simulink model "PX02s"  (R2015b)
settings: Solver=VariableStepAuto  StartTime=0.0  StopTime=10.0  RelTol=1e-3
libraries: fl_lib x10, nesl_utility x3
settings Model: Creator=xmax1946  LastModifiedBy=xmax1946

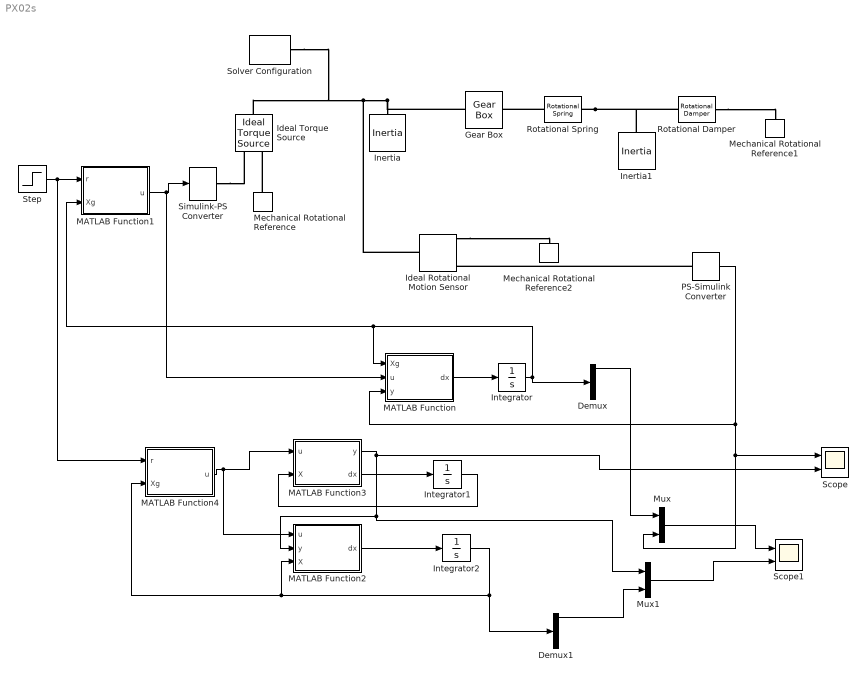
== system PX02s ==
  Demux : Demux
  Demux1 : Demux
  Gear Box : fl_lib/Mechanical/Mechanisms/Gear Box  ratio=100/30  t_in_specify=off  t_in_priority=None  t_in=0 N*m  t_out_specify=off  t_out_priority=None  t_out=0 N*m
  Ideal Rotational Motion Sensor : fl_lib/Mechanical/Mechanical Sensors/Ideal Rotational Motion Sensor  offset=0 rad
  Ideal Torque Source : fl_lib/Mechanical/Mechanical Sources/Ideal Torque Source
  Inertia : fl_lib/Mechanical/Rotational Elements/Inertia  inertia=50 kg*m^2  w_specify=off  w_priority=None  w=0 rad/s  t_specify=off  t_priority=None  t=0 N*m
  Inertia1 : fl_lib/Mechanical/Rotational Elements/Inertia  inertia=100 kg*m^2  w_specify=off  w_priority=None  w=0 rad/s  t_specify=off  t_priority=None  t=0 N*m
  Integrator : Integrator  InitialCondition=[1;1;1;1]
  Integrator1 : Integrator  InitialCondition=[0;0;0;0]  IgnoreLimit=on
  Integrator2 : Integrator  InitialCondition=[1;1;1;1]
  MATLAB Function : MATLAB Function  TreatAsAtomicUnit=on
  MATLAB Function1 : MATLAB Function  TreatAsAtomicUnit=on
  MATLAB Function2 : MATLAB Function  TreatAsAtomicUnit=on
  MATLAB Function3 : MATLAB Function  TreatAsAtomicUnit=on
  MATLAB Function4 : MATLAB Function  TreatAsAtomicUnit=on
  Mechanical Rotational Reference : fl_lib/Mechanical/Rotational Elements/Mechanical Rotational Reference
  Mechanical Rotational Reference1 : fl_lib/Mechanical/Rotational Elements/Mechanical Rotational Reference
  Mechanical Rotational Reference2 : fl_lib/Mechanical/Rotational Elements/Mechanical Rotational Reference
  Mux : Mux  Inputs=2
  Mux1 : Mux  Inputs=2
  PS-Simulink Converter : nesl_utility/PS-Simulink Converter  PhysicalDomain=network_engine_domain  SubClassName=ps_output  LeftPortType=input  RightPortType=output  PseudoPeriodic=off  Frequencies=[]  Unit=1  AffineConversion=off
  Rotational Damper : fl_lib/Mechanical/Rotational Elements/Rotational Damper  D=100 N*m/(rad/s)  w_specify=off  w_priority=None  w=0 rad/s  t_specify=off  t_priority=None  t=0 N*m
  Rotational Spring : fl_lib/Mechanical/Rotational Elements/Rotational Spring  spr_rate=100 N*m/rad  w_specify=off  w_priority=None  w=0 rad/s  t_specify=off  t_priority=None  t=0 N*m  phi_specify=off  phi_priority=None  phi=0 rad
  Scope : Scope  NumInputPorts=2
  Scope1 : Scope  NumInputPorts=2
  Simulink-PS Converter : nesl_utility/Simulink-PS Converter  PhysicalDomain=network_engine_domain  SubClassName=ps_input  LeftPortType=input  RightPortType=output  PseudoPeriodic=off  Frequencies=[]  NoiseDistribution=none  NoiseParameters=[]  Unit=1  AffineConversion=off  InputFiltering=off  SimscapeFilterOrder=1  InputFilterTimeConstant=0.001  UdotUserProvided=1
  Solver Configuration : nesl_utility/Solver Configuration  PhysicalDomain=network_engine_domain  SubClassName=solver  LeftPortType=input  RightPortType=generic  Accelerate=off  Tones=[]  Harmonics=[]  SimulateNoise=off  Profile=off  UseLocalSampling=off  EnableSwitchedLinearOptims=on  FrequencyDomain=off  UseCCode=off  RelTol=0.001  AbsTol=1e-06  MinStep=1e-09  ToWorkspace=off  RevertToSquareIcSolve=off  NumHomotopyIterations=100  PhasorMode=off  PhasorModeNumHarmonics=1  DoDC=off  ResidualTolerance=1e-09  UseLocalSolver=off  LocalSolverChoice=NE_BACKWARD_EULER_ADVANCER  LocalSolverSampleTime=0.001  DoFixedCost=off  MaxNonlinIter=3  MaxModeIter=2  LinearAlgebra=Sparse  DelaysMemoryBudget=1024  AutomaticFiltering=on  FilteringTimeConstant=0.001
  Step : Step  SampleTime=0
  wires:
  MATLAB Function/1(dx) -> Integrator/1
  Integrator/1 -> MATLAB Function1/2(Xg), MATLAB Function/1(Xg), Demux/1
  PS-Simulink Converter/1 -> Mux/2, Scope/1, MATLAB Function/3(y)
  ? -> ?
  Step/1 -> MATLAB Function4/1(r), MATLAB Function1/1(r)
  MATLAB Function1/1(u) -> MATLAB Function/2(u), Simulink-PS Converter/1
  MATLAB Function4/1(u) -> MATLAB Function2/1(u), MATLAB Function3/1(u)
  MATLAB Function2/1(dx) -> Integrator2/1
  MATLAB Function3/2(dx) -> Integrator1/1
  Integrator1/1 -> MATLAB Function3/2(X)
  Integrator2/1 -> Demux1/1, MATLAB Function4/2(Xg), MATLAB Function2/3(X)
  MATLAB Function3/1(y) -> Scope/2, Mux1/1, MATLAB Function2/2(y)
  Demux/1 -> Mux/1
  Mux/1 -> Scope1/1
  Demux1/1 -> Mux1/2
  Mux1/1 -> Scope1/2
  connections:
  Inertia/LConn1 -- Gear Box/LConn1 -- Ideal Rotational Motion Sensor/LConn1 -- Ideal Torque Source/LConn1 -- Solver Configuration/RConn1
  Rotational Spring/RConn1 -- Inertia1/LConn1 -- Rotational Damper/LConn1
  Rotational Damper/RConn1 -- Mechanical Rotational Reference1/LConn1
  Simulink-PS Converter/RConn1 -- Ideal Torque Source/RConn1
  Mechanical Rotational Reference/LConn1 -- Ideal Torque Source/RConn2
  Rotational Spring/LConn1 -- Gear Box/RConn1
  PS-Simulink Converter/LConn1 -- Ideal Rotational Motion Sensor/RConn3
  Ideal Rotational Motion Sensor/RConn1 -- Mechanical Rotational Reference2/LConn1

== matlab function PX02s/MATLAB Function1 ==
  data: r input; u output; Xg input
function u = fcn(r,Xg)
K=[3991,750,8809,8050];
u=r-K*Xg;

== matlab function PX02s/MATLAB Function ==
  data: dx output; Xg input; u input; y input
function dx  = fss(Xg,u,y)
A=[0,1,0,0
   -9/50,0,9/50,0
   0,0,0,1
   1,0,-1,-1];
B=[0;1/50;0;0];
C=[1,0,0,0];
L=[31;351.82;9250;11551];
dx=A*Xg+B*u+L*(y-C*Xg);

== matlab function PX02s/MATLAB Function2 ==
  data: u input; y input; X input; dx output
function dx  = fcn(u,y,X)
A=[0,1,0,0
   -9/50,0,9/50,0
   0,0,0,1
   1,0,-1,-1];
B=[0;1/50;0;0];
C=[1,0,0,0];
L=[31;351.82;9250;11551];
dx=A*X+B*u+(L*(y-C*X));

== matlab function PX02s/MATLAB Function3 ==
  data: u input; y output; X input; dx output
function [y,dx] = fcn(u,X)
A=[0,1,0,0
   -9/50,0,9/50,0
   0,0,0,1
   1,0,-1,-1];
B=[0;1/50;0;0];
C=[1,0,0,0];

dx=A*X+B*u;
y=C*X;

== matlab function PX02s/MATLAB Function4 ==
  data: r input; u output; Xg input
function u = fcn(r,Xg)
K=[3991,750,8809,8050];
u=r-K*Xg;
